simulink model "versao2"  (R2022a)
settings: Solver=VariableStepAuto  StartTime=0.0  StopTime=100  MaxStep=1e-5  RelTol=1e-3
libraries: simulink x1
settings Model: Creator=juan-  LastModifiedBy=juan-

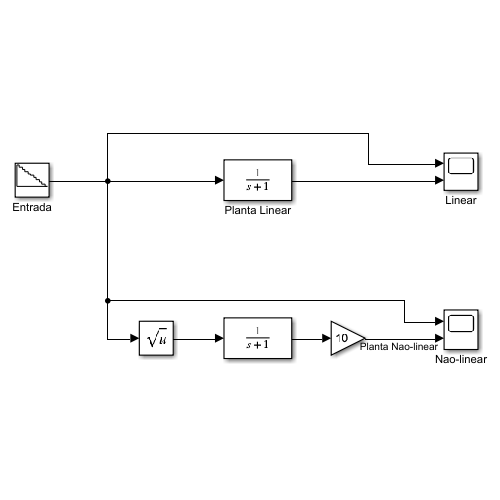
[thumbnail: Simulink's stored preview of the top-level diagram]
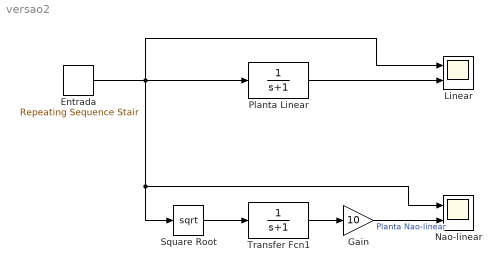
== system versao2 ==
  Entrada : simulink/Sources/Repeating Sequence Stair  OutValues=[100 90 80 70 60 50 40 30 20 10 0].'  tsamp=10  OutMin=[]  OutMax=[]  OutDataTypeStr=double  OutputDataTypeScalingMode=double  OutDataType=fixdt(0,8)  ConRadixGroup=Best Precision: Vector-wise  OutScaling=2^-12
  Gain : Gain  Gain=10
  Linear : Scope  NumInputPorts=2
  Nao-linear : Scope  NumInputPorts=2
  Planta Linear : TransferFcn  Denominator=[1 1]
  Square Root : Sqrt
  Transfer Fcn1 : TransferFcn  Denominator=[1 1]
  wires:
  Square Root/1 -> Transfer Fcn1/1
  Entrada/1 -> Linear/1, Nao-linear/1, Square Root/1, Planta Linear/1
  Planta Linear/1 -> Linear/2
  Transfer Fcn1/1 -> Gain/1
  Gain/1 -> Nao-linear/2  "Planta Nao-linear"
